simulink model "KitticopterSimulation"  (R2022a)
settings: Solver=VariableStepAuto  StartTime=0.0  StopTime=500  RelTol=1e-3
libraries: cstblocks x1, simulink x1
settings Model: Creator=User  LastModifiedBy=User

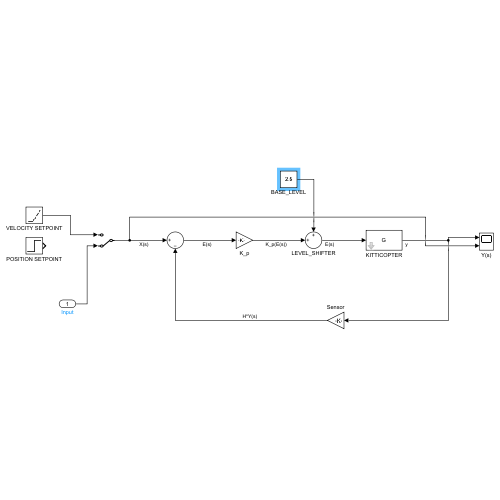
[thumbnail: Simulink's stored preview of the top-level diagram]
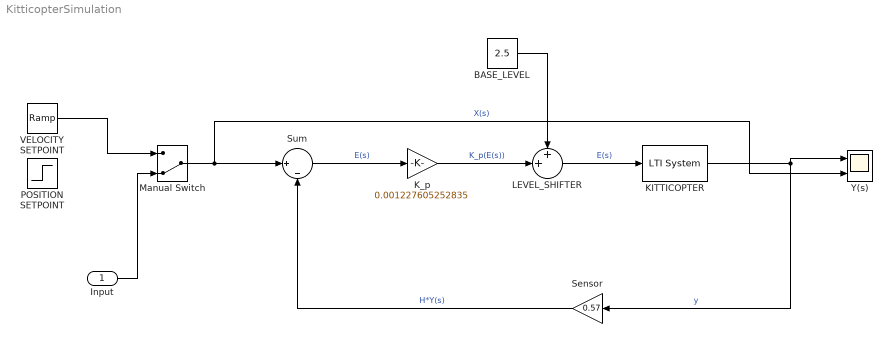
== system KitticopterSimulation ==
  Input : Inport
  BASE_LEVEL : Constant  Value=2.5  SampleTime=-1
  KITTICOPTER : cstblocks/LTI System  sys=G  IC=[]
  K_p : Gain  Gain=0.001227605252835
  LEVEL_SHIFTER : Sum  Inputs=++|
  Manual Switch : ManualSwitch  CurrentSetting=0
  POSITION SETPOINT : Step  SampleTime=0
  Sensor : Gain  Gain=0.57
  Sum : Sum  Inputs=||+|-
  VELOCITY SETPOINT : simulink/Sources/Ramp  slope=1  start=0  InitialOutput=0
  Y(s) : Scope  NumInputPorts=2
  wires:
  Sum/1 -> K_p/1  "E(s)"
  KITTICOPTER/1 -> Y(s)/1, Sensor/1  "y"
  Sensor/1 -> Sum/2  "H*Y(s)"
  Manual Switch/1 -> Y(s)/2, Sum/1  "X(s)"
  VELOCITY SETPOINT/1 -> Manual Switch/1
  K_p/1 -> LEVEL_SHIFTER/2  "K_p(E(s))"
  LEVEL_SHIFTER/1 -> KITTICOPTER/1  "E(s)"
  BASE_LEVEL/1 -> LEVEL_SHIFTER/1
  Input/1 -> Manual Switch/2
